simulink model "figura_3"  (R2021b)
settings: Solver=ode23t  StartTime=0.0  StopTime=0.1  RelTol=1e-5
libraries: spsGroundLib x2, spsCurrentMeasurementLib x2, spsPowerLib x2, spsVoltageMeasurementLib x2, spsThreePhaseSourceLib x1, spsThreePhaseSeriesRLCBranchLib x1, spspowerguiLib x1
settings Model: Creator=alanp  LastModifiedBy=luang
settings SolverCC: AlgebraicLoopSolver=TrustRegion
settings DebuggingCC: SFMachineParentedDataDiag=warning

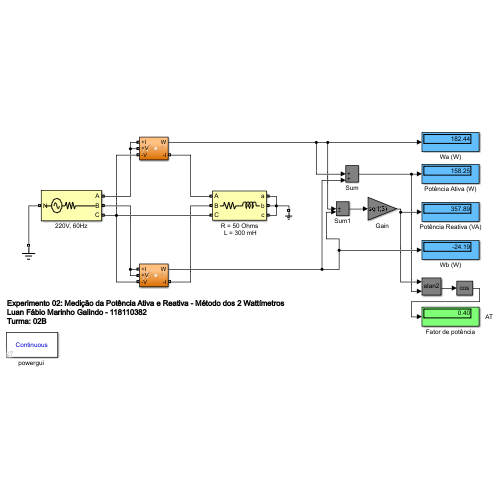
[thumbnail: Simulink's stored preview of the top-level diagram]
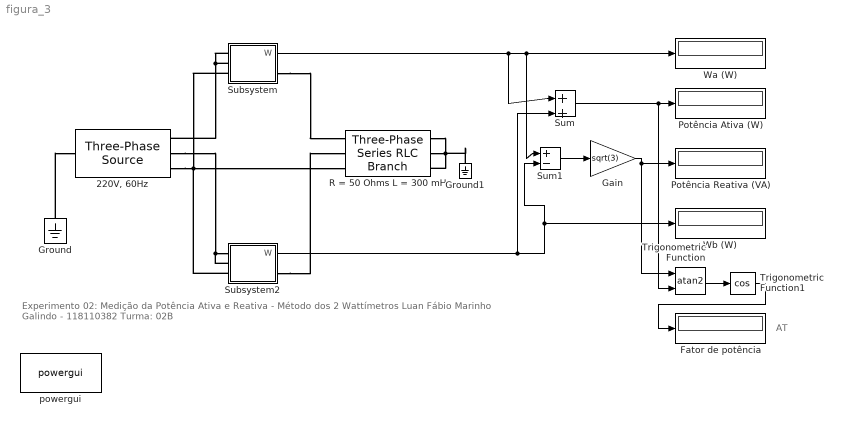
== system figura_3 ==
  note: AT
  note: Experimento 02: Medição da Potência Ativa e Reativa - Método dos 2 Wattímetros
      | Luan Fábio Marinho Galindo - 118110382
      | Turma: 02B
  "220V, 60Hz" : spsThreePhaseSourceLib/Three-Phase Source  InternalConnection=Yn  VoltagePhases=off  Voltage=220  PhaseAngle=90  Voltage_phases=[25e3 25e3 25e3]/sqrt(3)  PhaseAngles_phases=[0 -120 +120]  Frequency=60  NonIdealSource=on  SpecifyImpedance=off  Resistance=0.001  Inductance=0  ShortCircuitLevel=100e6  BaseVoltage=25e3  XRratio=7  BusType=swing  Pref=10e3  Qref=0  Prefabc=[10e3, 10e3, 10e3]  Qrefabc=[0, 0, 0]  Qmin=-inf  Qmax=inf
  Fator de potência : Display
      settings: Format=bank
  Gain : Gain  Gain=sqrt(3)
  Ground : spsGroundLib/Ground  LConnTagsString=a
  Ground1 : spsGroundLib/Ground  LConnTagsString=a
  Potência Ativa (W) : Display
      settings: Format=bank
  Potência Reativa (VA) : Display
      settings: Format=bank
  R = 50 Ohms L = 300 mH : spsThreePhaseSeriesRLCBranchLib/Three-Phase Series RLC Branch  LConnTagsString=A|B|C  RConnTagsString=A|B|C  BranchType=RL  Resistance=50  Inductance=300e-3  Capacitance=0  Measurements=None
  Subsystem : Subsystem
  Subsystem2 : Subsystem
  Sum : Sum  Inputs=|++
  Sum1 : Sum  Inputs=|+-
  Trigonometric Function : Trigonometry  Operator=atan2
  Trigonometric Function1 : Trigonometry  Operator=cos
  Wa (W) : Display
      settings: Format=bank
  Wb (W) : Display
      settings: Format=bank
  "powergui " : spspowerguiLib/powergui  Priority=1  SimulationMode=Continuous  SampleTime=50e-6  frequency=60  Iterations=50  frequencyindice=60  Pbase=100e6  ErrMax=1e-4  UnitsV=kV  UnitsW=MW  buscounter=0  FunctionMessages=off  echomessages=off  EnableUseOfTLC=off  CurrentSourceSwitches=off  DisableSnubberDevices=off  DisableRonSwitches=off  DisableVfSwitches=off  DisplayEquations=off  AutomaticDiscreteSolvers=off  SolverType=Tustin/Backward Euler (TBE)  Interpol=off  ExternalGateDelay=off  methode=off  Ts=100  x0status=blocks  SPID=on  SwTol=0  HookPort=off  NonlinearTolerance=1e-4  nMaxIteration=100  ContinueOnMaxIteration=off  RestoreLinks=warning  ResistiveCurrentMeasurement=off  Frange=[0:2:500]  Ylog=off  Xlog=on  ShowGrid=off  save=off  variable=ZData  structure=0  ZoomFFT=off  StartTime=0.0  cycles=1  DisplayStyle=1  fundamental=60  FreqAxis=off  MaxFrequency=1000  frequencyindicesteady=1  RmsSteady=1  display=off
  wires:
  Subsystem/1(W) -> Wa (W)/1, Sum1/1, Sum/1
  Subsystem2/1(W) -> Sum1/2, Wb (W)/1, Sum/2
  Sum/1 -> Trigonometric Function/2, Potência Ativa (W)/1
  Sum1/1 -> Gain/1
  Gain/1 -> Trigonometric Function/1, Potência Reativa (VA)/1
  Trigonometric Function/1 -> Trigonometric Function1/1
  Trigonometric Function1/1 -> Fator de potência/1
  connections:
  Ground/LConn1 -- "220V, 60Hz"/LConn1
  "220V, 60Hz"/RConn3 -- R = 50 Ohms L = 300 mH/LConn3 -- Subsystem/LConn3 -- Subsystem2/LConn3
  R = 50 Ohms L = 300 mH/RConn1 -- Ground1/LConn1 -- R = 50 Ohms L = 300 mH/RConn2 -- R = 50 Ohms L = 300 mH/RConn3
  Subsystem/RConn1 -- R = 50 Ohms L = 300 mH/LConn1
  Subsystem/LConn1 -- Subsystem/LConn2 -- "220V, 60Hz"/RConn1
  "220V, 60Hz"/RConn2 -- Subsystem2/LConn2 -- Subsystem2/LConn1
  Subsystem2/RConn1 -- R = 50 Ohms L = 300 mH/LConn2

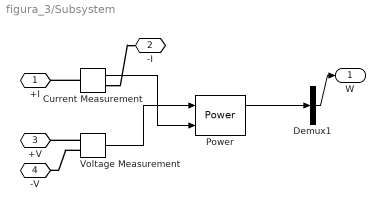
== system figura_3/Subsystem ==
  Current Measurement : spsCurrentMeasurementLib/Current Measurement  PhasorSimulation=off  OutputType=Complex  PSBequivalent=0
  Demux1 : Demux  Outputs=1
  Power : spsPowerLib/Power  Freq=60  Vinit=[1, 0]  Iinit=[1, 0]  Ts=0
      settings: SourceProductBaseCode=PS
  Voltage Measurement : spsVoltageMeasurementLib/Voltage Measurement  PhasorSimulation=off  OutputType=Complex  PSBequivalent=0
  +I : PMIOPort  Side=Left
  -I : PMIOPort  Port=2  Side=Right
  +V : PMIOPort  Port=3  Side=Left
  -V : PMIOPort  Port=4  Side=Left
  W : Outport
  wires:
  Current Measurement/1 -> Power/2
  Power/1 -> Demux1/1
  Demux1/1 -> W/1
  Voltage Measurement/1 -> Power/1
  connections:
  Voltage Measurement/LConn1 -- +V/RConn1
  Voltage Measurement/LConn2 -- -V/RConn1
  Current Measurement/LConn1 -- +I/RConn1
  Current Measurement/RConn1 -- -I/RConn1

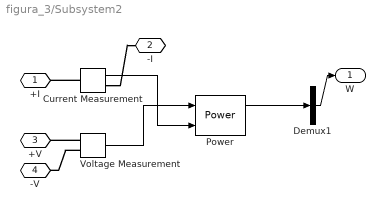
== system figura_3/Subsystem2 ==
  Current Measurement : spsCurrentMeasurementLib/Current Measurement  PhasorSimulation=off  OutputType=Complex  PSBequivalent=0
  Demux1 : Demux  Outputs=1
  Power : spsPowerLib/Power  Freq=60  Vinit=[1, 0]  Iinit=[1, 0]  Ts=0
      settings: SourceProductBaseCode=PS
  Voltage Measurement : spsVoltageMeasurementLib/Voltage Measurement  PhasorSimulation=off  OutputType=Complex  PSBequivalent=0
  +I : PMIOPort  Side=Left
  -I : PMIOPort  Port=2  Side=Right
  +V : PMIOPort  Port=3  Side=Left
  -V : PMIOPort  Port=4  Side=Left
  W : Outport
  wires:
  Current Measurement/1 -> Power/2
  Power/1 -> Demux1/1
  Demux1/1 -> W/1
  Voltage Measurement/1 -> Power/1
  connections:
  Voltage Measurement/LConn1 -- +V/RConn1
  Voltage Measurement/LConn2 -- -V/RConn1
  Current Measurement/LConn1 -- +I/RConn1
  Current Measurement/RConn1 -- -I/RConn1
